simulink model "simulator"  (R2022b)
settings: Solver=FixedStepAuto  StartTime=0.0  StopTime=1800  FixedStep=1/7000  RelTol=1e-7
undefined symbols (not defined in the file): simdb
libraries: sim_lib x40, simulink_extras x15, matrix_library x9, simulink x1
(part 1 of 3)
settings Model: SimulationMode=accelerator  Creator=David  LastModifiedBy=David

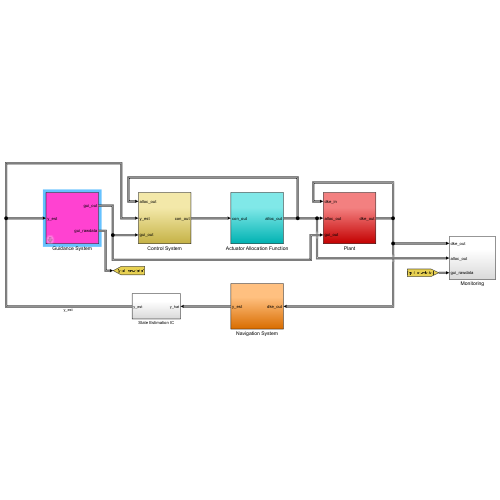
[thumbnail: Simulink's stored preview of the top-level diagram]
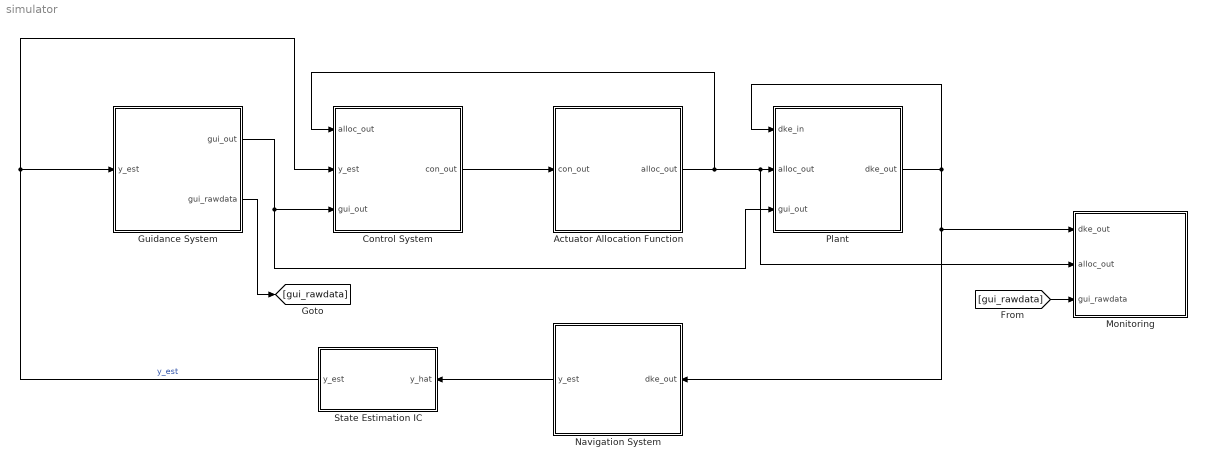
== system simulator ==
  Actuator Allocation Function : Subsystem
  Control System : Subsystem
  Guidance System : Subsystem  mask{gui=simdb.gui}
      mask prompts: gui "Guidance Parameters"
  Monitoring : Subsystem
  Navigation System : Subsystem
  Plant : Subsystem
  State Estimation IC : Subsystem
  wires:
  State Estimation IC/1(y_est) -> Control System/2(y_est), Guidance System/1(y_est)  "y_est"
  Navigation System/1(y_est) -> State Estimation IC/1(y_hat)
  Plant/1(dke_out) -> Navigation System/1(dke_out), Monitoring/1(dke_out), Plant/1(dke_in)
  Actuator Allocation Function/1(alloc_out) -> Plant/2(alloc_out), Monitoring/2(alloc_out), Control System/1(alloc_out)
  Guidance System/1(gui_out) -> Plant/3(gui_out), Control System/3(gui_out)
  Control System/1(con_out) -> Actuator Allocation Function/1(con_out)
  Guidance System/2(gui_rawdata) -> [gui_rawdata]
  [gui_rawdata] -> Monitoring/3(gui_rawdata)

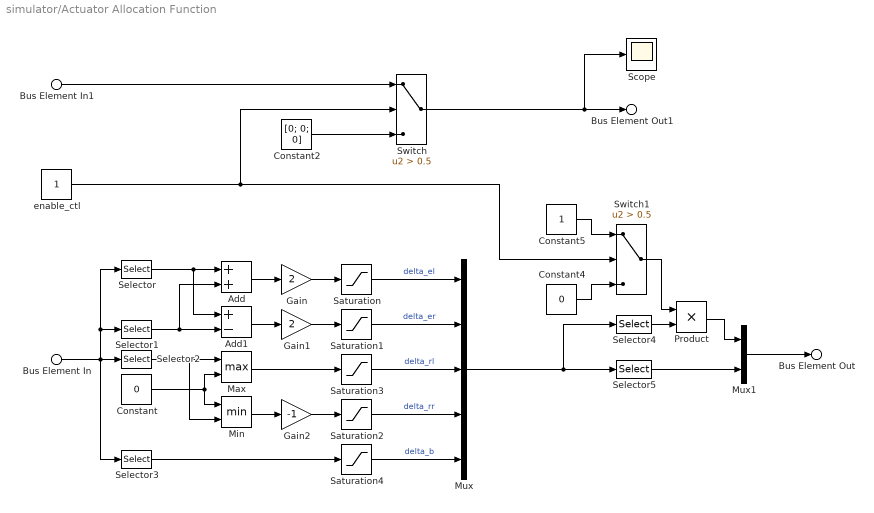
== system simulator/Actuator Allocation Function ==
  Bus Element In : Inport  PortName=con_out  Element=sc_delta_ae_cmd
  Bus Element In1 : Inport  PortName=con_out  Element=sc_rcs_tor_bod_cmd
  Add : Sum
  Add1 : Sum  Inputs=+-
  Constant : Constant  Value=0
  Constant2 : Constant  Value=[0; 0; 0]
  Constant4 : Constant  Value=0
  Constant5 : Constant
  Gain : Gain  Gain=2
  Gain1 : Gain  Gain=2
  Gain2 : Gain  Gain=-1
  Max : MinMax  Function=max  Inputs=2
  Min : MinMax  Inputs=2
  Mux : Mux  Inputs=5
  Mux1 : Mux  Inputs=2
  Product : Product
  Saturation : Saturate  UpperLimit=simdb.sc.delta_e_bounds(2)  LowerLimit=simdb.sc.delta_e_bounds(1)
  Saturation1 : Saturate  UpperLimit=simdb.sc.delta_e_bounds(2)  LowerLimit=simdb.sc.delta_e_bounds(1)
  Saturation2 : Saturate  UpperLimit=simdb.sc.delta_r_bounds(2)  LowerLimit=simdb.sc.delta_r_bounds(1)
  Saturation3 : Saturate  UpperLimit=simdb.sc.delta_r_bounds(2)  LowerLimit=simdb.sc.delta_r_bounds(1)
  Saturation4 : Saturate  UpperLimit=simdb.sc.delta_b_bounds(2)  LowerLimit=simdb.sc.delta_b_bounds(1)
  Scope : Scope
  Selector : Selector  InputPortWidth=4  IndexOptions=Index vector (dialog)  Indices=[1]  OutputSizes=1
  Selector1 : Selector  InputPortWidth=4  IndexOptions=Index vector (dialog)  Indices=[2]  OutputSizes=1
  Selector2 : Selector  InputPortWidth=4  IndexOptions=Index vector (dialog)  Indices=[3]  OutputSizes=1
  Selector3 : Selector  InputPortWidth=4  IndexOptions=Index vector (dialog)  Indices=[4]  OutputSizes=1
  Selector4 : Selector  InputPortWidth=5  IndexOptions=Index vector (dialog)  Indices=1:4  OutputSizes=1
  Selector5 : Selector  InputPortWidth=5  IndexOptions=Index vector (dialog)  Indices=[5]  OutputSizes=1
  Switch : Switch  Criteria=u2 > Threshold  Threshold=0.5  SaturateOnIntegerOverflow=off  InputSameDT=off
  Switch1 : Switch  Criteria=u2 > Threshold  Threshold=0.5  SaturateOnIntegerOverflow=off  InputSameDT=off
  enable_ctl : Constant
  Bus Element Out : Outport  PortName=alloc_out  Element=delta_ae_cmd
  Bus Element Out1 : Outport  PortName=alloc_out  Element=T_cmd
  wires:
  Bus Element In/1 -> Selector/1, Selector1/1, Selector3/1, Selector2/1
  Selector1/1 -> Add/2, Add1/2
  Selector/1 -> Add1/1, Add/1
  Add/1 -> Gain/1
  Add1/1 -> Gain1/1
  Gain/1 -> Saturation/1
  Gain1/1 -> Saturation1/1
  Selector2/1 -> Min/2, Max/1
  Constant/1 -> Max/2, Min/1
  Min/1 -> Gain2/1
  Gain2/1 -> Saturation2/1
  Max/1 -> Saturation3/1
  Selector3/1 -> Saturation4/1
  Saturation3/1 -> Mux/3  "delta_rl"
  Saturation/1 -> Mux/1  "delta_el"
  Saturation1/1 -> Mux/2  "delta_er"
  Saturation2/1 -> Mux/4  "delta_rr"
  Saturation4/1 -> Mux/5  "delta_b"
  Mux/1 -> Selector5/1, Selector4/1
  enable_ctl/1 -> Switch/2, Switch1/2
  Bus Element In1/1 -> Switch/1
  Constant2/1 -> Switch/3
  Constant4/1 -> Switch1/3
  Constant5/1 -> Switch1/1
  Selector4/1 -> Product/2
  Switch1/1 -> Product/1
  Product/1 -> Mux1/1
  Selector5/1 -> Mux1/2
  Mux1/1 -> Bus Element Out/1
  Switch/1 -> Scope/1, Bus Element Out1/1

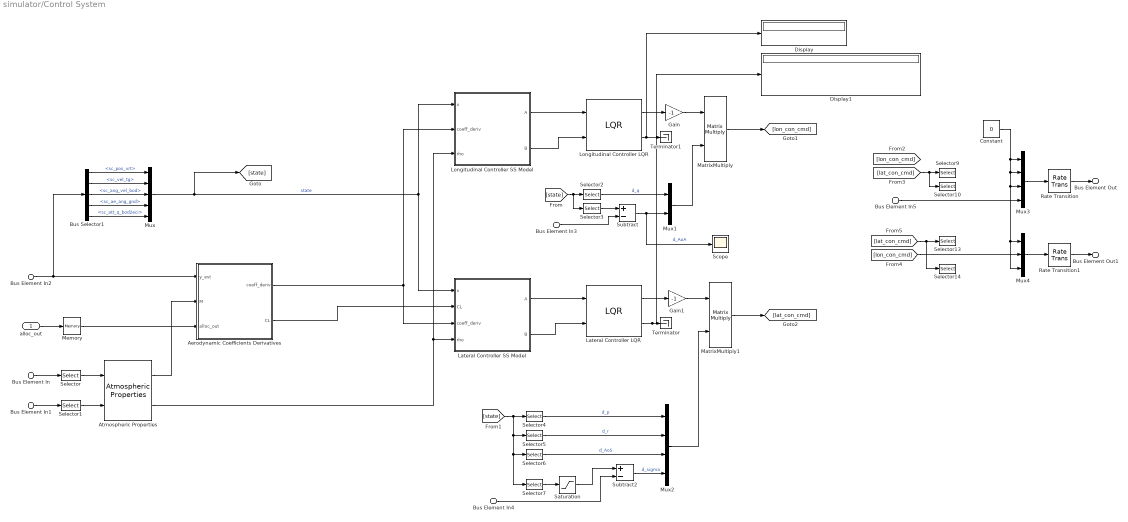
== system simulator/Control System ==
  alloc_out : Inport
  Bus Element In2 : Inport  Port=2  PortName=y_est
  Bus Element In : Inport  Port=2  PortName=y_est  Element=sc_vel_tg
  Bus Element In1 : Inport  Port=2  PortName=y_est  Element=sc_pos_vrt
  Bus Element In3 : Inport  Port=3  PortName=gui_out  Element=AoA_cmd
  Bus Element In5 : Inport  Port=3  PortName=gui_out  Element=delta_b_cmd
  Bus Element In4 : Inport  Port=3  PortName=gui_out  Element=bank_ang_cmd
  Aerodynamic Coefficients Derivatives : Subsystem
  Atmospheric Properties : sim_lib/Atmospheric Properties  Rp=simdb.env.Rp  Rg=simdb.env.Rg  gamma=simdb.env.gamma  h_base=simdb.env.h_base  T_base=simdb.env.T_base  rho_base=simdb.env.rho_base
  Bus Selector1 : BusSelector  OutputSignals=sc_pos_vrt,sc_vel_tg,sc_ang_vel_bod,sc_ae_ang_gnd,sc_att_q_bod2eci
  Constant : Constant  Value=0
  Display : Display
  Display1 : Display
  Gain : Gain  Gain=-1
  Gain1 : Gain  Gain=-1
  Lateral Controller LQR : sim_lib/LQR  Q=simdb.ctl.Q_lat  R=simdb.ctl.R_lat  X0=eye(4)
  Lateral Controller SS Model : MATLAB Function  TreatAsAtomicUnit=on  mask{S=simdb.sc.Sref, b=simdb.sc.bref, Ixx=simdb.sc.I(1,1), Izz=simdb.sc.I(3,3), m=simdb.sc.m, mu=simdb.env.mu}
      mask prompts: S "Reference area [m^2]:"; b "Lateral reference length [m]:"; Ixx "Inertia, x axis [kg*m^2]:"; Izz "Inertia, z axis [kg*m^2]:"; m "Mass [kg]:"; mu "Gravitational parameter [m^3/s^2]:"
  Longitudinal Controller LQR : sim_lib/LQR  Q=simdb.ctl.Q_lon  R=simdb.ctl.R_lon  X0=eye(2)
  Longitudinal Controller SS Model : MATLAB Function  TreatAsAtomicUnit=on  mask{S=simdb.sc.Sref, c=simdb.sc.cref, Iyy=simdb.sc.I(2,2), m=simdb.sc.m}
      mask prompts: S "Reference area [m^2]:"; c "Longitudinal reference length [m]:"; Iyy "Inertia, y axis [kg*m^2]:"; m "Mass [kg]:"
  MatrixMultiply : Product  Multiplication=Matrix(*)
  MatrixMultiply1 : Product  Multiplication=Matrix(*)
  Memory : Memory
  Mux : Mux  Inputs=5
  Mux1 : Mux  Inputs=2
  Mux2 : Mux
  Mux3 : Mux
  Mux4 : Mux  Inputs=3
  Rate Transition : RateTransition  InitialCondition=[0; 0; 0; 0]  OutPortSampleTime=simdb.ctl.tsamp
  Rate Transition1 : RateTransition  InitialCondition=[0; 0; 0]  OutPortSampleTime=simdb.ctl.tsamp
  Saturation : Saturate  UpperLimit=deg2rad(180)  LowerLimit=deg2rad(-180)
  Scope : Scope
  Selector : Selector  InputPortWidth=3  IndexOptions=Index vector (dialog)  Indices=[1]  OutputSizes=1
  Selector1 : Selector  InputPortWidth=3  IndexOptions=Index vector (dialog)  Indices=[1]  OutputSizes=1
  Selector10 : Selector  InputPortWidth=4  IndexOptions=Index vector (dialog)  Indices=[2]  OutputSizes=1
  Selector13 : Selector  InputPortWidth=4  IndexOptions=Index vector (dialog)  Indices=[3]  OutputSizes=1
  Selector14 : Selector  InputPortWidth=4  IndexOptions=Index vector (dialog)  Indices=[4]  OutputSizes=1
  Selector2 : Selector  InputPortWidth=16  IndexOptions=Index vector (dialog)  Indices=[8]  OutputSizes=1
  Selector3 : Selector  InputPortWidth=16  IndexOptions=Index vector (dialog)  Indices=[10]  OutputSizes=1
  Selector4 : Selector  InputPortWidth=16  IndexOptions=Index vector (dialog)  Indices=[7]  OutputSizes=1
  Selector5 : Selector  InputPortWidth=16  IndexOptions=Index vector (dialog)  Indices=[9]  OutputSizes=1
  Selector6 : Selector  InputPortWidth=16  IndexOptions=Index vector (dialog)  Indices=[9]  OutputSizes=1
  Selector7 : Selector  InputPortWidth=16  IndexOptions=Index vector (dialog)  Indices=[9]  OutputSizes=1
  Selector9 : Selector  InputPortWidth=4  IndexOptions=Index vector (dialog)  Indices=[1]  OutputSizes=1
  Subtract : Sum  Inputs=+-
  Subtract2 : Sum  Inputs=+-
  Terminator : Terminator
  Terminator1 : Terminator
  Bus Element Out : Outport  PortName=con_out  Element=sc_delta_ae_cmd
  Bus Element Out1 : Outport  PortName=con_out  Element=sc_rcs_tor_bod_cmd
  wires:
  Lateral Controller SS Model/1(A) -> Lateral Controller LQR/1
  Lateral Controller SS Model/2(B) -> Lateral Controller LQR/2
  Longitudinal Controller SS Model/1(A) -> Longitudinal Controller LQR/1
  Longitudinal Controller SS Model/2(B) -> Longitudinal Controller LQR/2
  alloc_out/1 -> Memory/1
  Memory/1 -> Aerodynamic Coefficients Derivatives/3(alloc_out)
  Selector/1 -> Atmospheric Properties/1
  Bus Element In/1 -> Selector/1
  Bus Element In1/1 -> Selector1/1
  Selector1/1 -> Atmospheric Properties/2
  Bus Element In2/1 -> Bus Selector1/1, Aerodynamic Coefficients Derivatives/1(y_est)
  Atmospheric Properties/1 -> Aerodynamic Coefficients Derivatives/2(M)
  Bus Selector1/3 -> Mux/3  "<sc_ang_vel_bod>"
  Bus Selector1/4 -> Mux/4  "<sc_ae_ang_gnd>"
  Bus Selector1/5 -> Mux/5  "<sc_att_q_bod2eci>"
  Bus Selector1/2 -> Mux/2  "<sc_vel_tg>"
  Bus Selector1/1 -> Mux/1  "<sc_pos_vrt>"
  Mux/1 -> [state], Longitudinal Controller SS Model/1(x), Lateral Controller SS Model/1(x)  "state"
  Aerodynamic Coefficients Derivatives/1(coeff_deriv) -> Longitudinal Controller SS Model/2(coeff_deriv), Lateral Controller SS Model/3(coeff_deriv)
  Atmospheric Properties/2 -> Lateral Controller SS Model/4(rho), Longitudinal Controller SS Model/3(rho)
  Lateral Controller LQR/2 -> Terminator/1, Display1/1
  Longitudinal Controller LQR/2 -> Terminator1/1, Display/1
  [state] -> Selector3/1, Selector2/1
  Selector3/1 -> Subtract/1
  Bus Element In3/1 -> Subtract/2
  Subtract/1 -> Scope/1, Mux1/2  "d_AoA"
  Selector2/1 -> Mux1/1  "d_q"
  Longitudinal Controller LQR/1 -> Gain/1
  Mux1/1 -> MatrixMultiply/2
  Gain/1 -> MatrixMultiply/1
  Lateral Controller LQR/1 -> Gain1/1
  Gain1/1 -> MatrixMultiply1/1
  [state] -> Selector7/1, Selector6/1, Selector5/1, Selector4/1
  Selector5/1 -> Mux2/2  "d_r"
  Selector4/1 -> Mux2/1  "d_p"
  Subtract2/1 -> Mux2/4  "d_sigma"
  Selector7/1 -> Saturation/1
  Selector6/1 -> Mux2/3  "d_AoS"
  Mux3/1 -> Rate Transition/1
  MatrixMultiply1/1 -> [lat_con_cmd]
  [lat_con_cmd] -> Selector10/1, Selector9/1
  Bus Element In5/1 -> Mux3/4
  Mux4/1 -> Rate Transition1/1
  [lat_con_cmd] -> Selector14/1, Selector13/1
  Aerodynamic Coefficients Derivatives/2(CL) -> Lateral Controller SS Model/2(CL)
  Mux2/1 -> MatrixMultiply1/2
  Rate Transition/1 -> Bus Element Out/1
  Rate Transition1/1 -> Bus Element Out1/1
  Bus Element In4/1 -> Subtract2/2
  Saturation/1 -> Subtract2/1
  Constant/1 -> Mux3/1, Mux4/3, Mux4/1, Mux3/3, Mux3/2
  MatrixMultiply/1 -> [lon_con_cmd]
  [lon_con_cmd] -> Mux4/2

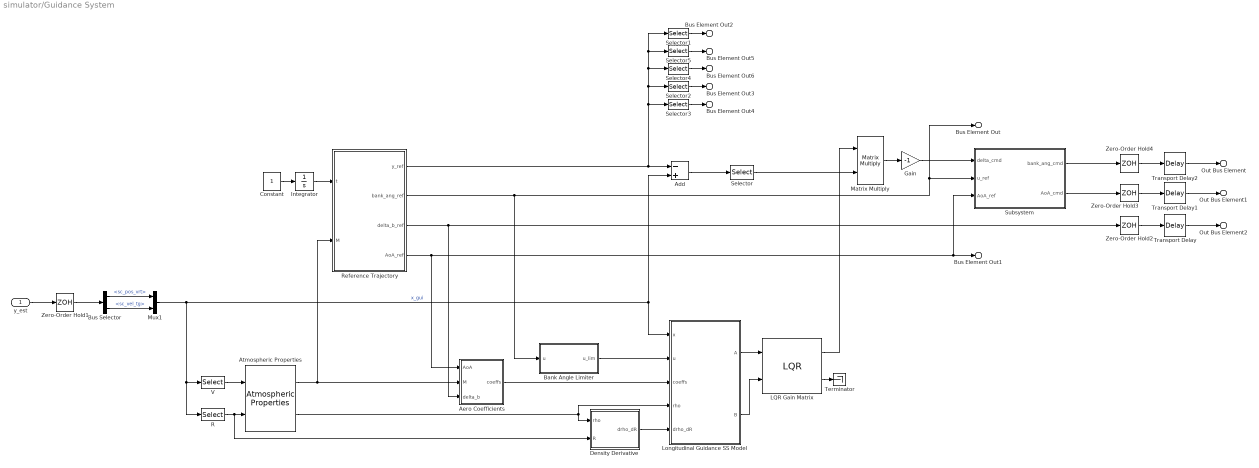
== system simulator/Guidance System ==
  y_est : Inport
  Add : Sum  Inputs=-+
  Aero Coefficients : Subsystem
  Atmospheric Properties : sim_lib/Atmospheric Properties  Rp=simdb.env.Rp  Rg=simdb.env.Rg  gamma=simdb.env.gamma  h_base=simdb.env.h_base  T_base=simdb.env.T_base  rho_base=simdb.env.rho_base
  Bank Angle Limiter : Subsystem
  Bus Selector : BusSelector  OutputSignals=sc_pos_vrt,sc_vel_tg
  Constant : Constant
  Density Derivative : Subsystem
  Gain : Gain  Gain=-1
  Integrator : Integrator  InitialCondition=1
  LQR Gain Matrix : sim_lib/LQR  Q=gui.Q  R=gui.R  X0=eye(3)
  Longitudinal Guidance SS Model : MATLAB Function  TreatAsAtomicUnit=on  mask{S=simdb.sc.Sref, m=simdb.sc.m, mu=simdb.env.mu}
      mask prompts: S "Reference area"; m "Spacecraft mass"; mu "Gravitational constant"
  Matrix Multiply : Product  Multiplication=Matrix(*)
  Mux1 : Mux  Inputs=2
  R : Selector  InputPortWidth=6  IndexOptions=Index vector (dialog)  Indices=[1]  OutputSizes=1
  Reference Trajectory : Subsystem
  Selector : Selector  InputPortWidth=6  IndexOptions=Index vector (dialog)  Indices=[1 4 5]  OutputSizes=1
  Selector1 : Selector  InputPortWidth=6  IndexOptions=Index vector (dialog)  Indices=1  OutputSizes=1
  Selector2 : Selector  InputPortWidth=6  IndexOptions=Index vector (dialog)  Indices=4  OutputSizes=1
  Selector3 : Selector  InputPortWidth=6  IndexOptions=Index vector (dialog)  Indices=5  OutputSizes=1
  Selector4 : Selector  InputPortWidth=6  IndexOptions=Index vector (dialog)  Indices=3  OutputSizes=1
  Selector5 : Selector  InputPortWidth=6  IndexOptions=Index vector (dialog)  Indices=2  OutputSizes=1
  Subsystem : Subsystem
  Terminator : Terminator
  Transport Delay : TransportDelay  DelayTime=gui.delay  BufferSize=4096
  Transport Delay1 : TransportDelay  DelayTime=gui.delay  InitialOutput=deg2rad(-40)  BufferSize=4096
  Transport Delay2 : TransportDelay  DelayTime=gui.delay  InitialOutput=deg2rad(-165)  BufferSize=4096
  V : Selector  InputPortWidth=6  IndexOptions=Index vector (dialog)  Indices=[4]  OutputSizes=1
  Zero-Order Hold{1..4} (4 alike) : ZeroOrderHold  SampleTime=gui.tsample
  Out Bus Element : Outport  PortName=gui_out  Element=bank_ang_cmd
  Out Bus Element2 : Outport  PortName=gui_out  Element=delta_b_cmd
  Out Bus Element1 : Outport  PortName=gui_out  Element=AoA_cmd
  Bus Element Out : Outport  Port=2  PortName=gui_rawdata  Element=bank_ang_ref
  Bus Element Out1 : Outport  Port=2  PortName=gui_rawdata  Element=AoA_ref
  Bus Element Out2 : Outport  Port=2  PortName=gui_rawdata  Element=R_ref
  Bus Element Out3 : Outport  Port=2  PortName=gui_rawdata  Element=V_ref
  Bus Element Out4 : Outport  Port=2  PortName=gui_rawdata  Element=gamma_ref
  Bus Element Out5 : Outport  Port=2  PortName=gui_rawdata  Element=tau_ref
  Bus Element Out6 : Outport  Port=2  PortName=gui_rawdata  Element=delta_ref
  wires:
  y_est/1 -> Zero-Order Hold1/1
  Mux1/1 -> V/1, R/1, Longitudinal Guidance SS Model/1(x), Add/2  "x_gui"
  Zero-Order Hold2/1 -> Transport Delay/1
  Constant/1 -> Integrator/1
  Longitudinal Guidance SS Model/1(A) -> LQR Gain Matrix/1
  Matrix Multiply/1 -> Gain/1
  Reference Trajectory/3(delta_b_ref) -> Aero Coefficients/3(delta_b), Zero-Order Hold2/1
  Reference Trajectory/2(bank_ang_ref) -> Bank Angle Limiter/1(u), Bus Element Out/1, Subsystem/2(u_ref)
  Reference Trajectory/4(AoA_ref) -> Aero Coefficients/1(AoA), Subsystem/3(AoA_ref), Bus Element Out1/1
  Integrator/1 -> Reference Trajectory/1(t)
  Selector/1 -> Matrix Multiply/2
  Add/1 -> Selector/1
  Atmospheric Properties/2 -> Density Derivative/1(rho), Longitudinal Guidance SS Model/4(rho)
  Atmospheric Properties/1 -> Aero Coefficients/2(M), Reference Trajectory/2(M)
  V/1 -> Atmospheric Properties/1
  R/1 -> Density Derivative/2(R), Atmospheric Properties/2
  Density Derivative/1(drho_dR) -> Longitudinal Guidance SS Model/5(drho_dR)
  Longitudinal Guidance SS Model/2(B) -> LQR Gain Matrix/2
  LQR Gain Matrix/1 -> Matrix Multiply/1
  LQR Gain Matrix/2 -> Terminator/1
  Zero-Order Hold1/1 -> Bus Selector/1
  Bus Selector/1 -> Mux1/1  "<sc_pos_vrt>"
  Bus Selector/2 -> Mux1/2  "<sc_vel_tg>"
  Transport Delay/1 -> Out Bus Element2/1
  Zero-Order Hold4/1 -> Transport Delay2/1
  Transport Delay2/1 -> Out Bus Element/1
  Aero Coefficients/1(coeffs) -> Longitudinal Guidance SS Model/3(coeffs)
  Gain/1 -> Subsystem/1(delta_cmd)
  Subsystem/1(bank_ang_cmd) -> Zero-Order Hold4/1
  Transport Delay1/1 -> Out Bus Element1/1
  Zero-Order Hold3/1 -> Transport Delay1/1
  Subsystem/2(AoA_cmd) -> Zero-Order Hold3/1
  Bank Angle Limiter/1(u_lim) -> Longitudinal Guidance SS Model/2(u)
  Selector1/1 -> Bus Element Out2/1
  Selector2/1 -> Bus Element Out3/1
  Selector3/1 -> Bus Element Out4/1
  Selector4/1 -> Bus Element Out6/1
  Reference Trajectory/1(y_ref) -> Selector4/1, Selector5/1, Selector1/1, Selector2/1, Selector3/1, Add/1
  Selector5/1 -> Bus Element Out5/1

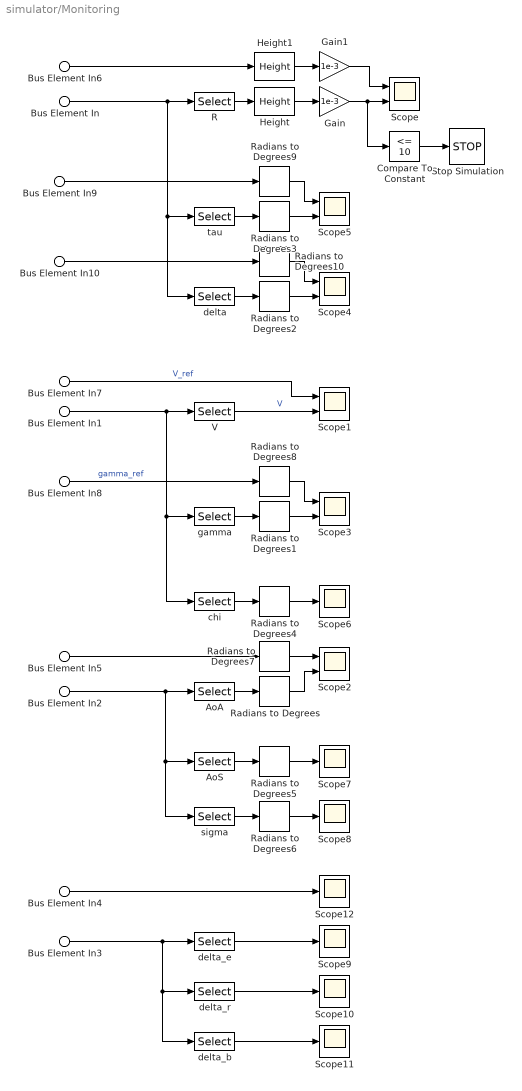
== system simulator/Monitoring ==
  Bus Element In : Inport  PortName=dke_out  Element=sc_pos_vrt
  Bus Element In1 : Inport  PortName=dke_out  Element=sc_vel_tg
  Bus Element In2 : Inport  PortName=dke_out  Element=sc_ae_ang_gnd
  Bus Element In4 : Inport  PortName=dke_out  Element=sc_att_q_bod2eci
  Bus Element In3 : Inport  Port=2  PortName=alloc_out  Element=delta_ae_cmd
  Bus Element In5 : Inport  Port=3  PortName=gui_rawdata  Element=AoA_ref
  Bus Element In6 : Inport  Port=3  PortName=gui_rawdata  Element=R_ref
  Bus Element In7 : Inport  Port=3  PortName=gui_rawdata  Element=V_ref
  Bus Element In8 : Inport  Port=3  PortName=gui_rawdata  Element=gamma_ref
  Bus Element In10 : Inport  Port=3  PortName=gui_rawdata  Element=delta_ref
  Bus Element In9 : Inport  Port=3  PortName=gui_rawdata  Element=tau_ref
  AoA : Selector  InputPortWidth=3  IndexOptions=Index vector (dialog)  Indices=[1]  OutputSizes=1
  AoS : Selector  InputPortWidth=3  IndexOptions=Index vector (dialog)  Indices=[2]  OutputSizes=1
  Compare To Constant : simulink/Logic and Bit Operations/Compare To Constant  relop=<=  const=10  OutDataTypeStr=boolean
  Gain : Gain  Gain=1e-3
  Gain1 : Gain  Gain=1e-3
  Height : sim_lib/Height  Rp=simdb.env.Rp
  Height1 : sim_lib/Height  Rp=simdb.env.Rp
  R : Selector  InputPortWidth=3  IndexOptions=Index vector (dialog)  Indices=[1]  OutputSizes=1
  Radians to Degrees{,1..10} (11 alike) : simulink_extras/Transformations/Radians to Degrees
  Scope{,1..5} (6 alike) : Scope  NumInputPorts=2
  Scope{6..12} (7 alike) : Scope
  Stop Simulation : Stop
  V : Selector  InputPortWidth=3  IndexOptions=Index vector (dialog)  Indices=[1]  OutputSizes=1
  chi : Selector  InputPortWidth=3  IndexOptions=Index vector (dialog)  Indices=[3]  OutputSizes=1
  delta : Selector  InputPortWidth=3  IndexOptions=Index vector (dialog)  Indices=[3]  OutputSizes=1
  delta_b : Selector  InputPortWidth=5  IndexOptions=Index vector (dialog)  Indices=[5]  OutputSizes=1
  delta_e : Selector  InputPortWidth=5  IndexOptions=Index vector (dialog)  Indices=[1 2]  OutputSizes=1
  delta_r : Selector  InputPortWidth=5  IndexOptions=Index vector (dialog)  Indices=[3 4]  OutputSizes=1
  gamma : Selector  InputPortWidth=3  IndexOptions=Index vector (dialog)  Indices=[2]  OutputSizes=1
  sigma : Selector  InputPortWidth=3  IndexOptions=Index vector (dialog)  Indices=[3]  OutputSizes=1
  tau : Selector  InputPortWidth=3  IndexOptions=Index vector (dialog)  Indices=[2]  OutputSizes=1
  wires:
  R/1 -> Height/1
  AoA/1 -> Radians to Degrees/1
  gamma/1 -> Radians to Degrees1/1
  Height/1 -> Gain/1
  Gain/1 -> Scope/2, Compare To Constant/1
  Compare To Constant/1 -> Stop Simulation/1
  chi/1 -> Radians to Degrees4/1
  Radians to Degrees4/1 -> Scope6/1
  tau/1 -> Radians to Degrees3/1
  delta/1 -> Radians to Degrees2/1
  Bus Element In/1 -> delta/1, tau/1, R/1
  Bus Element In1/1 -> chi/1, gamma/1, V/1
  Bus Element In2/1 -> sigma/1, AoS/1, AoA/1
  Radians to Degrees5/1 -> Scope7/1
  AoS/1 -> Radians to Degrees5/1
  Radians to Degrees6/1 -> Scope8/1
  sigma/1 -> Radians to Degrees6/1
  Bus Element In3/1 -> delta_b/1, delta_r/1, delta_e/1
  delta_e/1 -> Scope9/1
  delta_r/1 -> Scope10/1
  delta_b/1 -> Scope11/1
  Bus Element In4/1 -> Scope12/1
  Bus Element In5/1 -> Radians to Degrees7/1
  Radians to Degrees7/1 -> Scope2/1
  Radians to Degrees/1 -> Scope2/2
  Height1/1 -> Gain1/1
  Bus Element In6/1 -> Height1/1
  Gain1/1 -> Scope/1
  V/1 -> Scope1/2  "V"
  Bus Element In7/1 -> Scope1/1  "V_ref"
  Bus Element In8/1 -> Radians to Degrees8/1  "gamma_ref"
  Radians to Degrees8/1 -> Scope3/1
  Radians to Degrees1/1 -> Scope3/2
  Radians to Degrees3/1 -> Scope5/2
  Bus Element In9/1 -> Radians to Degrees9/1
  Radians to Degrees2/1 -> Scope4/2
  Bus Element In10/1 -> Radians to Degrees10/1
  Radians to Degrees9/1 -> Scope5/1
  Radians to Degrees10/1 -> Scope4/1

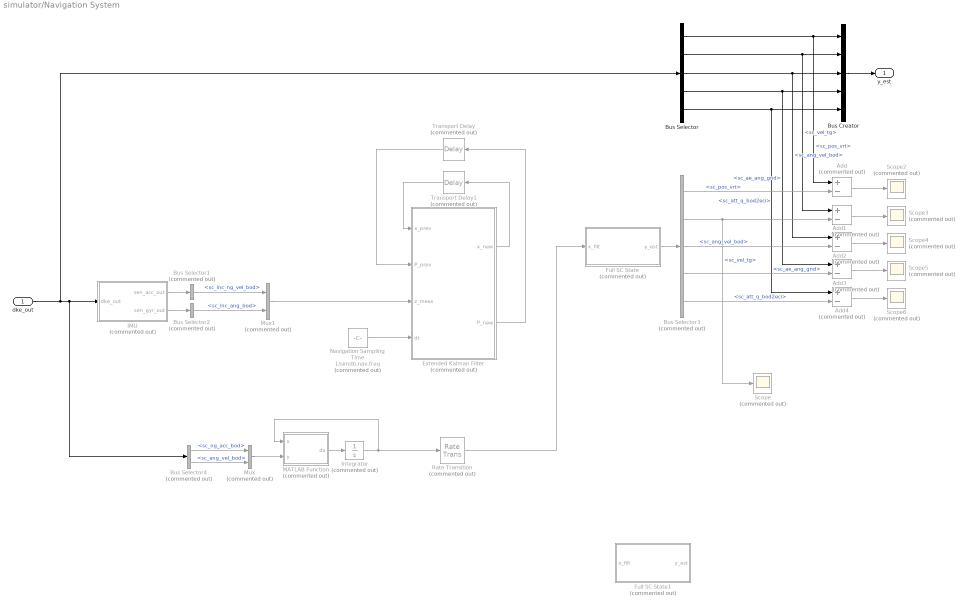
== system simulator/Navigation System ==
  dke_out : Inport
  Add{,1..4} (5 alike) : Sum  Commented=on  Inputs=+-
  Bus Creator : BusCreator  Inputs=5
  Bus Selector : BusSelector  OutputSignals=sc_pos_vrt,sc_vel_tg,sc_ang_vel_bod,sc_ae_ang_gnd,sc_att_q_bod2eci
  Bus Selector1 : BusSelector  Commented=on  OutputSignals=sc_inc_ng_vel_bod
  Bus Selector2 : BusSelector  Commented=on  OutputSignals=sc_inc_ang_bod
  Bus Selector3 : BusSelector  Commented=on  OutputSignals=sc_pos_vrt,sc_vel_tg,sc_ang_vel_bod,sc_ae_ang_gnd,sc_att_q_bod2eci
  Bus Selector4 : BusSelector  Commented=on  OutputSignals=sc_ng_acc_bod,sc_ang_vel_bod
  Extended Kalman Filter : Subsystem  Commented=on
  Full SC State : Subsystem  Commented=on
  Full SC State1 : Subsystem  Commented=on
  IMU : Subsystem  Commented=on  mask{gyr=simdb.gyr, acc=simdb.acc}
      mask prompts: gyr "GYR Parameters"; acc "ACC Parameters"
  Integrator : Integrator  Commented=on  InitialCondition=simdb.nav.x0
  MATLAB Function : MATLAB Function  Commented=on  TreatAsAtomicUnit=on  mask{mu=simdb.env.mu, K=simdb.nav.dq_K}
  Mux : Mux  Commented=on  Inputs=2
  Mux1 : Mux  Commented=on  Inputs=2
  Navigation Sampling Time : Constant  Commented=on  Value=1/simdb.nav.freq
  Rate Transition : RateTransition  Commented=on  InitialCondition=simdb.nav.x0  OutPortSampleTime=simdb.nav.tsamp
  Scope{,2..6} (6 alike) : Scope  Commented=on
  Transport Delay : TransportDelay  Commented=on  DelayTime=simdb.nav.tsamp  InitialOutput=simdb.nav.P0
  Transport Delay1 : TransportDelay  Commented=on  DelayTime=simdb.nav.tsamp  InitialOutput=simdb.nav.x0
  y_est : Outport
  wires:
  IMU/1(sen_acc_out) -> Bus Selector1/1
  IMU/2(sen_gyr_out) -> Bus Selector2/1
  Bus Selector1/1 -> Mux1/1  "<sc_inc_ng_vel_bod>"
  Bus Selector2/1 -> Mux1/2  "<sc_inc_ang_bod>"
  dke_out/1 -> Bus Selector/1, Bus Selector4/1, IMU/1(dke_out)
  Transport Delay/1 -> Extended Kalman Filter/2(P_prev)
  Extended Kalman Filter/2(P_new) -> Transport Delay/1
  Transport Delay1/1 -> Extended Kalman Filter/1(x_prev)
  Navigation Sampling Time/1 -> Extended Kalman Filter/4(dt)
  Mux1/1 -> Extended Kalman Filter/3(z_meas)
  Extended Kalman Filter/1(x_new) -> Transport Delay1/1
  Bus Selector/5 -> Add4/1, Bus Creator/5  "<sc_att_q_bod2eci>"
  Bus Selector/4 -> Add3/1, Bus Creator/4  "<sc_ae_ang_gnd>"
  Bus Selector/3 -> Add2/1, Bus Creator/3  "<sc_ang_vel_bod>"
  Bus Selector/2 -> Add1/1, Bus Creator/2  "<sc_vel_tg>"
  Bus Selector/1 -> Add/1, Bus Creator/1  "<sc_pos_vrt>"
  Bus Creator/1 -> y_est/1
  Full SC State/1(y_est) -> Bus Selector3/1
  Bus Selector3/1 -> Add/2  "<sc_pos_vrt>"
  Bus Selector3/2 -> Scope/1, Add1/2  "<sc_vel_tg>"
  Bus Selector3/5 -> Add4/2  "<sc_att_q_bod2eci>"
  Bus Selector3/4 -> Add3/2  "<sc_ae_ang_gnd>"
  Bus Selector3/3 -> Add2/2  "<sc_ang_vel_bod>"
  Add/1 -> Scope2/1
  Add1/1 -> Scope3/1
  Add2/1 -> Scope4/1
  Add3/1 -> Scope5/1
  Add4/1 -> Scope6/1
  MATLAB Function/1(dx) -> Integrator/1
  Integrator/1 -> Rate Transition/1, MATLAB Function/1(x)
  Bus Selector4/1 -> Mux/1  "<sc_ng_acc_bod>"
  Bus Selector4/2 -> Mux/2  "<sc_ang_vel_bod>"
  Mux/1 -> MATLAB Function/2(y)
  Rate Transition/1 -> Full SC State/1(x_filt)

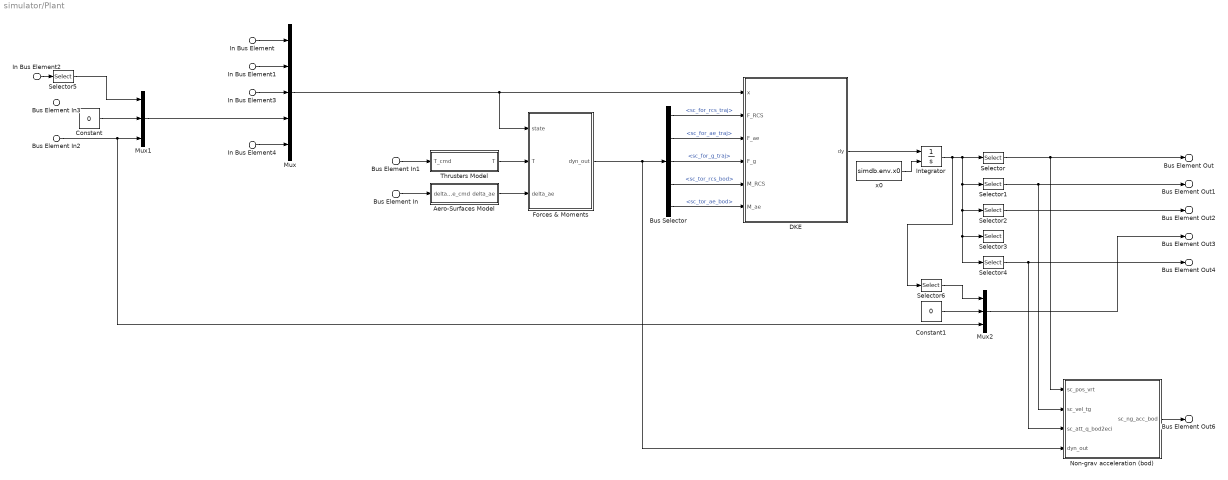
== system simulator/Plant ==
  In Bus Element : Inport  PortName=dke_in  Element=sc_pos_vrt
  In Bus Element1 : Inport  PortName=dke_in  Element=sc_vel_tg
  In Bus Element3 : Inport  PortName=dke_in  Element=sc_ang_vel_bod
  In Bus Element4 : Inport  PortName=dke_in  Element=sc_att_q_bod2eci
  In Bus Element2 : Inport  PortName=dke_in  Element=sc_ae_ang_gnd
  Bus Element In : Inport  Port=2  PortName=alloc_out  Element=delta_ae_cmd
  Bus Element In1 : Inport  Port=2  PortName=alloc_out  Element=T_cmd
  Bus Element In2 : Inport  Port=3  PortName=gui_out  Element=bank_ang_cmd
  Bus Element In3 : Inport  Port=3  PortName=gui_out  Element=AoA_cmd
  Aero-Surfaces Model : Subsystem
  Bus Selector : BusSelector  OutputSignals=sc_for_rcs_traj,sc_for_ae_traj,sc_for_g_traj,sc_tor_rcs_bod,sc_tor_ae_bod
  Constant : Constant  Value=0
  Constant1 : Constant  Value=0
  DKE : MATLAB Function  TreatAsAtomicUnit=on  mask{m=simdb.sc.m, omega_cb=simdb.env.omega_cb, I=simdb.sc.I}
  Forces & Moments : Subsystem
  Integrator : Integrator  InitialConditionSource=external
  Mux : Mux  Inputs=5
  Mux1 : Mux  Inputs=3
  Mux2 : Mux  Inputs=3
  Non-grav acceleration (bod) : Subsystem
  Selector : Selector  InputPortWidth=16  IndexOptions=Index vector (dialog)  Indices=[1 2 3]  OutputSizes=1
  Selector1 : Selector  InputPortWidth=16  IndexOptions=Index vector (dialog)  Indices=[4 5 6]  OutputSizes=1
  Selector2 : Selector  InputPortWidth=16  IndexOptions=Index vector (dialog)  Indices=[7 8 9]  OutputSizes=1
  Selector3 : Selector  InputPortWidth=16  IndexOptions=Index vector (dialog)  Indices=[10 11 12]  OutputSizes=1
  Selector4 : Selector  InputPortWidth=16  IndexOptions=Index vector (dialog)  Indices=[13 14 15 16]  OutputSizes=1
  Selector5 : Selector  InputPortWidth=3  IndexOptions=Index vector (dialog)  Indices=1  OutputSizes=1
  Selector6 : Selector  InputPortWidth=16  IndexOptions=Index vector (dialog)  Indices=10  OutputSizes=1
  Thrusters Model : Subsystem
  x0 : Constant  Value=simdb.env.x0
  Bus Element Out : Outport  PortName=dke_out  Element=sc_pos_vrt
  Bus Element Out1 : Outport  PortName=dke_out  Element=sc_vel_tg
  Bus Element Out2 : Outport  PortName=dke_out  Element=sc_ang_vel_bod
  Bus Element Out3 : Outport  PortName=dke_out  Element=sc_ae_ang_gnd
  Bus Element Out4 : Outport  PortName=dke_out  Element=sc_att_q_bod2eci
  Bus Element Out6 : Outport  PortName=dke_out  Element=sc_ng_acc_bod
  wires:
  Thrusters Model/1(T) -> Forces & Moments/2(T)
  Aero-Surfaces Model/1(delta_ae) -> Forces & Moments/3(delta_ae)
  Mux/1 -> Forces & Moments/1(state), DKE/1(x)
  DKE/1(dy) -> Integrator/1
  x0/1 -> Integrator/2
  Selector/1 -> Bus Element Out/1, Non-grav acceleration (bod)/1(sc_pos_vrt)
  Selector1/1 -> Bus Element Out1/1, Non-grav acceleration (bod)/2(sc_vel_tg)
  Selector2/1 -> Bus Element Out2/1
  Selector4/1 -> Bus Element Out4/1, Non-grav acceleration (bod)/3(sc_att_q_bod2eci)
  Integrator/1 -> Selector6/1, Selector4/1, Selector3/1, Selector2/1, Selector1/1, Selector/1
  Forces & Moments/1(dyn_out) -> Non-grav acceleration (bod)/4(dyn_out), Bus Selector/1
  Bus Selector/1 -> DKE/2(F_RCS)  "<sc_for_rcs_traj>"
  Bus Selector/2 -> DKE/3(F_ae)  "<sc_for_ae_traj>"
  Bus Selector/3 -> DKE/4(F_g)  "<sc_for_g_traj>"
  Bus Selector/4 -> DKE/5(M_RCS)  "<sc_tor_rcs_bod>"
  Bus Selector/5 -> DKE/6(M_ae)  "<sc_tor_ae_bod>"
  Non-grav acceleration (bod)/1(sc_ng_acc_bod) -> Bus Element Out6/1
  In Bus Element/1 -> Mux/1
  In Bus Element1/1 -> Mux/2
  In Bus Element4/1 -> Mux/5
  Bus Element In1/1 -> Thrusters Model/1(T_cmd)
  In Bus Element2/1 -> Selector5/1
  Constant/1 -> Mux1/2
  Bus Element In2/1 -> Mux2/3, Mux1/3
  Bus Element In/1 -> Aero-Surfaces Model/1(delta_ae_cmd)
  Constant1/1 -> Mux2/2
  Mux2/1 -> Bus Element Out3/1
  Mux1/1 -> Mux/4
  In Bus Element3/1 -> Mux/3
  Selector6/1 -> Mux2/1
  Selector5/1 -> Mux1/1

== system simulator/State Estimation IC ==
  y_hat : Inport
  Bus Creator : BusCreator  Inputs=5
  Bus Selector : BusSelector  OutputSignals=sc_pos_vrt,sc_vel_tg,sc_ang_vel_bod,sc_ae_ang_gnd,sc_att_q_bod2eci
  IC : InitialCondition  Value=simdb.nav.sc_pos_vrt_init
  IC1 : InitialCondition  Value=simdb.nav.sc_vel_tg_init
  IC2 : InitialCondition  Value=simdb.nav.sc_ang_vel_bod_init
  IC3 : InitialCondition  Value=simdb.nav.sc_ae_ang_gnd_init
  IC4 : InitialCondition  Value=simdb.nav.sc_att_q_bod2eci_init
  y_est : Outport
  wires:
  Bus Selector/3 -> IC2/1  "<sc_ang_vel_bod>"
  Bus Selector/1 -> IC/1  "<sc_pos_vrt>"
  IC4/1 -> Bus Creator/5  "sc_att_q_bod2eci"
  Bus Selector/2 -> IC1/1  "<sc_vel_tg>"
  Bus Selector/4 -> IC3/1  "<sc_ae_ang_gnd>"
  Bus Selector/5 -> IC4/1  "<sc_att_q_bod2eci>"
  Bus Creator/1 -> y_est/1
  IC/1 -> Bus Creator/1  "sc_pos_vrt"
  IC3/1 -> Bus Creator/4  "sc_ae_ang_gnd"
  IC1/1 -> Bus Creator/2  "sc_vel_tg"
  IC2/1 -> Bus Creator/3  "sc_ang_vel_bod"
  y_hat/1 -> Bus Selector/1

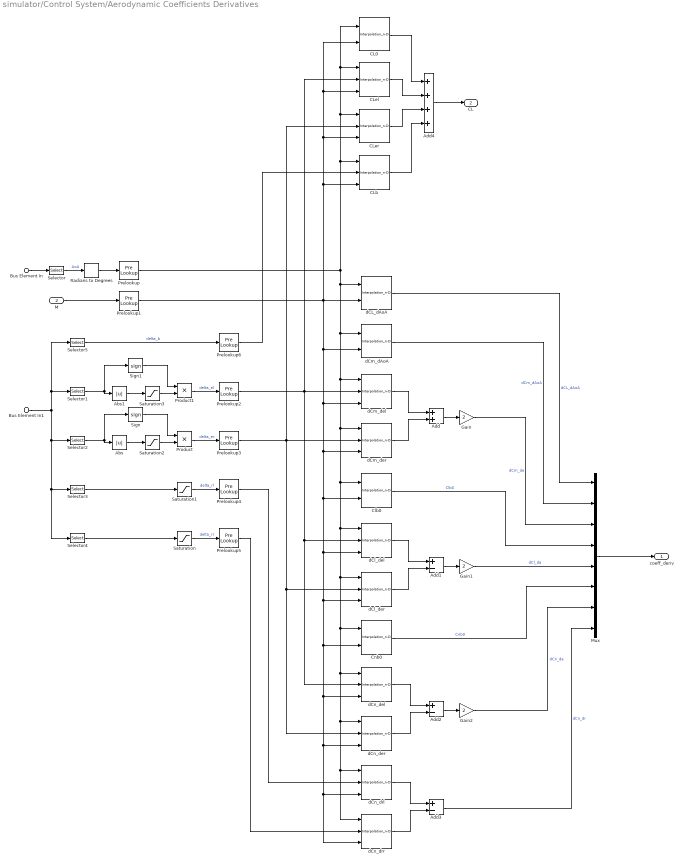
== system simulator/Control System/Aerodynamic Coefficients Derivatives ==
  Bus Element In : Inport  PortName=y_est  Element=sc_ae_ang_gnd
  M : Inport  Port=2
  Bus Element In1 : Inport  Port=3  PortName=alloc_out  Element=delta_ae_cmd
  Abs : Abs  SaturateOnIntegerOverflow=off
  Abs1 : Abs  SaturateOnIntegerOverflow=off
  Add : Sum
  Add1 : Sum  Inputs=+-
  Add2 : Sum  Inputs=+-
  Add3 : Sum  Inputs=+-
  Add4 : Sum  Inputs=++++
  CL0 : Interpolation_n-D  Table=simdb.aero.CL0  RequireIndexFractionAsBus=on  RemoveProtectionIndex=on  InternalRulePriority=Speed
      settings: InputPortMap=u0,u1
  CLb : Interpolation_n-D  NumberOfTableDimensions=3  Table=simdb.aero.CLb  RequireIndexFractionAsBus=on  RemoveProtectionIndex=on  InternalRulePriority=Speed
      settings: InputPortMap=u0,u1,u2
  CLel : Interpolation_n-D  NumberOfTableDimensions=3  Table=simdb.aero.CLel  RequireIndexFractionAsBus=on  RemoveProtectionIndex=on  InternalRulePriority=Speed
      settings: InputPortMap=u0,u1,u2
  CLer : Interpolation_n-D  NumberOfTableDimensions=3  Table=simdb.aero.CLel  RequireIndexFractionAsBus=on  RemoveProtectionIndex=on  InternalRulePriority=Speed
      settings: InputPortMap=u0,u1,u2
  Clb0 : Interpolation_n-D  Table=simdb.aero.Clb0  RequireIndexFractionAsBus=on  RemoveProtectionIndex=on  InternalRulePriority=Speed
      settings: InputPortMap=u0,u1
  Cnb0 : Interpolation_n-D  Table=simdb.aero.Cnb0  RequireIndexFractionAsBus=on  RemoveProtectionIndex=on  InternalRulePriority=Speed
      settings: InputPortMap=u0,u1
  Gain : Gain  Gain=2
  Gain1 : Gain  Gain=2
  Gain2 : Gain  Gain=2
  Mux : Mux  Inputs=8
  Prelookup : PreLookup  BreakpointsData=simdb.aero.AoA_table  OutputSelection=Index and fraction as bus  BeginIndexSearchUsingPreviousIndexResult=on  ExtrapMethod=Linear  RemoveProtectionInput=on
  Prelookup1 : PreLookup  BreakpointsData=simdb.aero.M_table  OutputSelection=Index and fraction as bus  BeginIndexSearchUsingPreviousIndexResult=on  ExtrapMethod=Linear  RemoveProtectionInput=on
  Prelookup2 : PreLookup  BreakpointsData=simdb.aero.delta_el_table  OutputSelection=Index and fraction as bus  BeginIndexSearchUsingPreviousIndexResult=on  ExtrapMethod=Linear  RemoveProtectionInput=on
  Prelookup3 : PreLookup  BreakpointsData=simdb.aero.delta_el_table  OutputSelection=Index and fraction as bus  BeginIndexSearchUsingPreviousIndexResult=on  ExtrapMethod=Linear  RemoveProtectionInput=on
  Prelookup4 : PreLookup  BreakpointsData=simdb.aero.delta_rl_table  OutputSelection=Index and fraction as bus  BeginIndexSearchUsingPreviousIndexResult=on  ExtrapMethod=Linear  RemoveProtectionInput=on
  Prelookup5 : PreLookup  BreakpointsData=simdb.aero.delta_rl_table  OutputSelection=Index and fraction as bus  BeginIndexSearchUsingPreviousIndexResult=on  ExtrapMethod=Linear  RemoveProtectionInput=on
  Prelookup6 : PreLookup  BreakpointsData=simdb.aero.delta_b_table  OutputSelection=Index and fraction as bus  BeginIndexSearchUsingPreviousIndexResult=on  ExtrapMethod=Linear  RemoveProtectionInput=on
  Product : Product
  Product1 : Product
  Radians to Degrees : simulink_extras/Transformations/Radians to Degrees
  Saturation : Saturate  UpperLimit=simdb.sc.delta_r_bounds(2)  LowerLimit=simdb.sc.delta_r_bounds(1)+1
  Saturation1 : Saturate  UpperLimit=simdb.sc.delta_r_bounds(2)  LowerLimit=simdb.sc.delta_r_bounds(1)+1
  Saturation2 : Saturate  UpperLimit=simdb.sc.delta_e_bounds(2)  LowerLimit=1
  Saturation3 : Saturate  UpperLimit=simdb.sc.delta_e_bounds(2)  LowerLimit=1
  Selector : Selector  InputPortWidth=3  IndexOptions=Index vector (dialog)  Indices=[1]  OutputSizes=1
  Selector1 : Selector  InputPortWidth=5  IndexOptions=Index vector (dialog)  Indices=[1]  OutputSizes=1
  Selector2 : Selector  InputPortWidth=5  IndexOptions=Index vector (dialog)  Indices=[2]  OutputSizes=1
  Selector3 : Selector  InputPortWidth=5  IndexOptions=Index vector (dialog)  Indices=[3]  OutputSizes=1
  Selector4 : Selector  InputPortWidth=5  IndexOptions=Index vector (dialog)  Indices=[4]  OutputSizes=1
  Selector5 : Selector  InputPortWidth=5  IndexOptions=Index vector (dialog)  Indices=[5]  OutputSizes=1
  Sign : Signum
  Sign1 : Signum
  dCL_dAoA : Interpolation_n-D  Table=simdb.aero.dCL_dAoA  RequireIndexFractionAsBus=on  RemoveProtectionIndex=on  InternalRulePriority=Speed
      settings: InputPortMap=u0,u1
  dCl_del : Interpolation_n-D  NumberOfTableDimensions=3  Table=simdb.aero.dCl_del  RequireIndexFractionAsBus=on  RemoveProtectionIndex=on  InternalRulePriority=Speed
      settings: InputPortMap=u0,u1,u2
  dCl_der : Interpolation_n-D  NumberOfTableDimensions=3  Table=simdb.aero.dCl_del  RequireIndexFractionAsBus=on  RemoveProtectionIndex=on  InternalRulePriority=Speed
      settings: InputPortMap=u0,u1,u2
  dCm_dAoA : Interpolation_n-D  Table=simdb.aero.dCm_dAoA  RequireIndexFractionAsBus=on  RemoveProtectionIndex=on  InternalRulePriority=Speed
      settings: InputPortMap=u0,u1
  dCm_del : Interpolation_n-D  NumberOfTableDimensions=3  Table=simdb.aero.dCm_del  RequireIndexFractionAsBus=on  RemoveProtectionIndex=on  InternalRulePriority=Speed
      settings: InputPortMap=u0,u1,u2
  dCm_der : Interpolation_n-D  NumberOfTableDimensions=3  Table=simdb.aero.dCm_del  RequireIndexFractionAsBus=on  RemoveProtectionIndex=on  InternalRulePriority=Speed
      settings: InputPortMap=u0,u1,u2
  dCn_del : Interpolation_n-D  NumberOfTableDimensions=3  Table=simdb.aero.dCn_del  RequireIndexFractionAsBus=on  RemoveProtectionIndex=on  InternalRulePriority=Speed
      settings: InputPortMap=u0,u1,u2
  dCn_der : Interpolation_n-D  NumberOfTableDimensions=3  Table=simdb.aero.dCn_del  RequireIndexFractionAsBus=on  RemoveProtectionIndex=on  InternalRulePriority=Speed
      settings: InputPortMap=u0,u1,u2
  dCn_drl : Interpolation_n-D  NumberOfTableDimensions=3  Table=simdb.aero.dCn_drl  RequireIndexFractionAsBus=on  RemoveProtectionIndex=on  InternalRulePriority=Speed
      settings: InputPortMap=u0,u1,u2
  dCn_drr : Interpolation_n-D  NumberOfTableDimensions=3  Table=simdb.aero.dCn_drl  RequireIndexFractionAsBus=on  RemoveProtectionIndex=on  InternalRulePriority=Speed
      settings: InputPortMap=u0,u1,u2
  coeff_deriv : Outport
  CL : Outport  Port=2
  wires:
  Bus Element In/1 -> Selector/1
  Selector/1 -> Radians to Degrees/1  "AoA"
  M/1 -> Prelookup1/1
  Prelookup/1 -> dCm_der/1, Clb0/1, dCl_der/1, Cnb0/1, dCn_der/1, dCn_drr/1, dCn_drl/1, dCn_del/1, dCl_del/1, dCm_del/1, dCm_dAoA/1, dCL_dAoA/1, CL0/1, CLel/1, CLer/1, CLb/1
  Prelookup1/1 -> dCm_der/3, Clb0/2, dCl_der/3, Cnb0/2, dCn_der/3, dCn_drr/3, dCn_drl/3, dCn_del/3, dCl_del/3, dCm_del/3, dCm_dAoA/2, CLer/3, CLel/3, CL0/2, CLb/3, dCL_dAoA/2
  Radians to Degrees/1 -> Prelookup/1
  Bus Element In1/1 -> Selector5/1, Selector1/1, Selector4/1, Selector3/1, Selector2/1
  Selector3/1 -> Saturation1/1
  Selector4/1 -> Saturation/1
  dCm_del/1 -> Add/1
  dCm_der/1 -> Add/2
  Add/1 -> Gain/1
  dCl_del/1 -> Add1/1
  dCl_der/1 -> Add1/2
  Add1/1 -> Gain1/1
  Add2/1 -> Gain2/1
  dCn_del/1 -> Add2/1
  dCn_der/1 -> Add2/2
  dCn_drl/1 -> Add3/1
  dCn_drr/1 -> Add3/2
  dCL_dAoA/1 -> Mux/1  "dCL_dAoA"
  dCm_dAoA/1 -> Mux/2  "dCm_dAoA"
  Gain/1 -> Mux/3  "dCm_de"
  Clb0/1 -> Mux/4  "Clb0"
  Gain1/1 -> Mux/5  "dCl_da"
  Cnb0/1 -> Mux/6  "Cnb0"
  Gain2/1 -> Mux/7  "dCn_da"
  Add3/1 -> Mux/8  "dCn_dr"
  Mux/1 -> coeff_deriv/1
  Add4/1 -> CL/1
  CLb/1 -> Add4/4
  CLel/1 -> Add4/2
  CL0/1 -> Add4/1
  CLer/1 -> Add4/3
  Selector5/1 -> Prelookup6/1  "delta_b"
  Prelookup6/1 -> CLb/2
  Prelookup5/1 -> dCn_drr/2
  Prelookup4/1 -> dCn_drl/2
  Prelookup3/1 -> dCn_der/2, dCl_der/2, CLer/2, dCm_der/2
  Prelookup2/1 -> dCl_del/2, dCn_del/2, CLel/2, dCm_del/2
  Abs1/1 -> Saturation3/1
  Selector1/1 -> Sign1/1, Abs1/1
  Sign1/1 -> Product1/1
  Saturation3/1 -> Product1/2
  Product1/1 -> Prelookup2/1  "delta_el"
  Sign/1 -> Product/1
  Saturation2/1 -> Product/2
  Abs/1 -> Saturation2/1
  Selector2/1 -> Sign/1, Abs/1
  Product/1 -> Prelookup3/1  "delta_er"
  Saturation1/1 -> Prelookup4/1  "delta_rl"
  Saturation/1 -> Prelookup5/1  "delta_rr"

== system simulator/Guidance System/Aero Coefficients ==
  AoA : Inport
  M : Inport  Port=2
  delta_b : Inport  Port=3
  Add : Sum
  Add1 : Sum
  AoA Table : PreLookup  BreakpointsData=simdb.aero.AoA_table  OutputSelection=Index and fraction as bus  BeginIndexSearchUsingPreviousIndexResult=on  ExtrapMethod=Linear  RemoveProtectionInput=on
  CD0 : Interpolation_n-D  Table=simdb.aero.CD0  RequireIndexFractionAsBus=on  RemoveProtectionIndex=on  InternalRulePriority=Speed
      settings: InputPortMap=u0,u1
  CDb : Interpolation_n-D  NumberOfTableDimensions=3  Table=simdb.aero.CDb  RequireIndexFractionAsBus=on  RemoveProtectionIndex=on  InternalRulePriority=Speed
      settings: InputPortMap=u0,u1,u2
  CL0 : Interpolation_n-D  Table=simdb.aero.CL0  RequireIndexFractionAsBus=on  RemoveProtectionIndex=on  InternalRulePriority=Speed
      settings: InputPortMap=u0,u1
  CLb : Interpolation_n-D  NumberOfTableDimensions=3  Table=simdb.aero.CLb  RequireIndexFractionAsBus=on  RemoveProtectionIndex=on  InternalRulePriority=Speed
      settings: InputPortMap=u0,u1,u2
  M Table : PreLookup  BreakpointsData=simdb.aero.M_table  OutputSelection=Index and fraction as bus  BeginIndexSearchUsingPreviousIndexResult=on  ExtrapMethod=Linear  RemoveProtectionInput=on
  Mux : Mux
  Radians to Degrees : simulink_extras/Transformations/Radians to Degrees
  dCD_dAoA : Interpolation_n-D  Table=simdb.aero.dCD_dAoA  RequireIndexFractionAsBus=on  RemoveProtectionIndex=on  InternalRulePriority=Speed
      settings: InputPortMap=u0,u1
  dCL_dAoA : Interpolation_n-D  Table=simdb.aero.dCL_dAoA  RequireIndexFractionAsBus=on  RemoveProtectionIndex=on  InternalRulePriority=Speed
      settings: InputPortMap=u0,u1
  delta_b Table : PreLookup  BreakpointsData=simdb.aero.delta_b_table  OutputSelection=Index and fraction as bus  BeginIndexSearchUsingPreviousIndexResult=on  ExtrapMethod=Linear  RemoveProtectionInput=on
  coeffs : Outport
  wires:
  Add/1 -> Mux/1  "CD"
  Add1/1 -> Mux/2  "CL"
  AoA/1 -> Radians to Degrees/1
  Radians to Degrees/1 -> AoA Table/1
  M/1 -> M Table/1
  delta_b/1 -> delta_b Table/1
  AoA Table/1 -> dCL_dAoA/1, dCD_dAoA/1, CLb/1, CDb/1, CL0/1, CD0/1
  delta_b Table/1 -> CDb/2, CLb/2
  M Table/1 -> CD0/2, dCL_dAoA/2, dCD_dAoA/2, CLb/3, CDb/3, CL0/2
  CD0/1 -> Add/1
  CDb/1 -> Add/2
  CL0/1 -> Add1/1
  CLb/1 -> Add1/2
  dCD_dAoA/1 -> Mux/3  "dCD_dAoA"
  dCL_dAoA/1 -> Mux/4  "dCL_dAoA"
  Mux/1 -> coeffs/1

== system simulator/Guidance System/Bank Angle Limiter ==
  u : Inport
  Abs : Abs  SaturateOnIntegerOverflow=off
  Product1 : Product
  Saturation : Saturate  UpperLimit=deg2rad(165)  LowerLimit=deg2rad(2)
  Sign : Signum
  u_lim : Outport
  wires:
  Abs/1 -> Saturation/1
  Saturation/1 -> Product1/2
  Sign/1 -> Product1/1
  u/1 -> Sign/1, Abs/1
  Product1/1 -> u_lim/1

== system simulator/Guidance System/Density Derivative ==
  rho : Inport
  R : Inport  Port=2
  Delay One Step : Delay  DelayLength=1
  Delay One Step1 : Delay  DelayLength=1
  Product : Product  Inputs=*/
  Sum : Sum  Inputs=|+-
  Sum1 : Sum  Inputs=|+-
  drho_dR : Outport
  wires:
  rho/1 -> Sum/1
  Sum/1 -> Product/1, Delay One Step/1
  Delay One Step1/1 -> Sum1/2
  Delay One Step/1 -> Sum/2
  Sum1/1 -> Product/2, Delay One Step1/1
  R/1 -> Sum1/1
  Product/1 -> drho_dR/1

== system simulator/Guidance System/Reference Trajectory ==
  t : Inport
  M : Inport  Port=2
  Ref Angle of Attack : MATLAB Function  TreatAsAtomicUnit=on
  Ref Bank Angle : Lookup_n-D  NumberOfTableDimensions=1  BreakpointsForDimension1=gui.t_gui  BreakpointsForDimension2=[1:3]  Table=gui.u_gui(1,:)  RemoveProtectionInput=on  InternalRulePriority=Speed  RndMeth=Simplest
  Ref Trajectory : Subsystem
  Ref body flap deflection : Lookup_n-D  NumberOfTableDimensions=1  BreakpointsForDimension1=gui.t_gui  BreakpointsForDimension2=[1:3]  Table=gui.u_gui(2,:)  RemoveProtectionInput=on  InternalRulePriority=Speed  RndMeth=Simplest
  y_ref : Outport
  bank_ang_ref : Outport  Port=2
  delta_b_ref : Outport  Port=3
  AoA_ref : Outport  Port=4
  wires:
  Ref body flap deflection/1 -> delta_b_ref/1
  t/1 -> Ref Trajectory/1(t), Ref body flap deflection/1, Ref Bank Angle/1
  Ref Angle of Attack/1(AoA) -> AoA_ref/1
  Ref Bank Angle/1 -> bank_ang_ref/1
  M/1 -> Ref Angle of Attack/1(M)
  Ref Trajectory/1(y_ref) -> y_ref/1

== system simulator/Guidance System/Subsystem ==
  delta_cmd : Inport
  u_ref : Inport  Port=2
  AoA_ref : Inport  Port=3
  Add : Sum
  Add1 : Sum
  Saturation : Saturate  UpperLimit=deg2rad(42.5)  LowerLimit=deg2rad(0)
  Saturation1 : Saturate  UpperLimit=deg2rad(170)  LowerLimit=-deg2rad(170)
  Selector : Selector  InputPortWidth=2  IndexOptions=Index vector (dialog)  Indices=2  OutputSizes=1
  Selector1 : Selector  InputPortWidth=2  IndexOptions=Index vector (dialog)  Indices=1  OutputSizes=1
  bank_ang_cmd : Outport
  AoA_cmd : Outport  Port=2
  wires:
  Add/1 -> Saturation1/1
  Selector/1 -> Add/2
  u_ref/1 -> Add/1
  delta_cmd/1 -> Selector/1, Selector1/1
  Selector1/1 -> Add1/1
  AoA_ref/1 -> Add1/2
  Add1/1 -> Saturation/1
  Saturation/1 -> AoA_cmd/1
  Saturation1/1 -> bank_ang_cmd/1

== system simulator/Navigation System/Extended Kalman Filter ==
  x_prev : Inport
  P_prev : Inport  Port=2
  z_meas : Inport  Port=3
  dt : Inport  Port=4
  Add : Sum
  Covariance Matrix Estimation : Subsystem
  Covariance Matrix Update : Subsystem
  Kalman Gain : Subsystem
  Matrix Multiply : Product  Multiplication=Matrix(*)
  Rate Transition : RateTransition  InitialCondition=simdb.nav.x0  OutPortSampleTime=simdb.nav.tsamp
  Rate Transition1 : RateTransition  InitialCondition=simdb.nav.P0  OutPortSampleTime=simdb.nav.tsamp
  Subtract : Sum  Inputs=+-
  estimation function : MATLAB Function  TreatAsAtomicUnit=on  mask{mu=simdb.env.mu, K=simdb.nav.dq_K}
      mask prompts: mu "Gravitational parameter [m^3/s^2]:"; K "dq integration gain:"
  estimation matrix : MATLAB Function  TreatAsAtomicUnit=on  mask{mu=simdb.env.mu}
      mask prompts: mu "Gravitational parameter [m^2/s^2]:"
  observation function : MATLAB Function  TreatAsAtomicUnit=on  mask{Ma=simdb.nav.Ma, Mo=simdb.nav.Mo}
      mask prompts: Ma "Acc Misalignment Matrix:"; Mo "Gyr Misalignment Matrix:"
  observation matrix : MATLAB Function  TreatAsAtomicUnit=on  mask{Ma=simdb.nav.Ma, Mo=simdb.nav.Mo}
      mask prompts: Ma "Acc Misalignment Matrix:"; Mo "Gyr Misalignment Matrix:"
  x_new : Outport
  P_new : Outport  Port=2
  wires:
  dt/1 -> observation function/2(dt), observation matrix/2(dt), estimation function/2(dt)
  x_prev/1 -> estimation matrix/1(x), estimation function/1(x)
  observation function/1(z) -> Subtract/2  "z_est"
  estimation function/1(x_est) -> Add/1, observation matrix/1(x), observation function/1(x)  "x_est"
  observation matrix/1(H) -> Covariance Matrix Update/2(H), Kalman Gain/1(H)
  Kalman Gain/1(K) -> Matrix Multiply/1, Covariance Matrix Update/1(K)
  z_meas/1 -> Subtract/1
  Subtract/1 -> Matrix Multiply/2
  Matrix Multiply/1 -> Add/2
  P_prev/1 -> Covariance Matrix Estimation/2(P_prev)
  Covariance Matrix Estimation/1(P_est) -> Covariance Matrix Update/3(P_est), Kalman Gain/2(P_est)
  Covariance Matrix Update/1(P_new) -> Rate Transition1/1
  Add/1 -> Rate Transition/1
  estimation matrix/1(F) -> Covariance Matrix Estimation/1(F)
  Rate Transition/1 -> x_new/1
  Rate Transition1/1 -> P_new/1

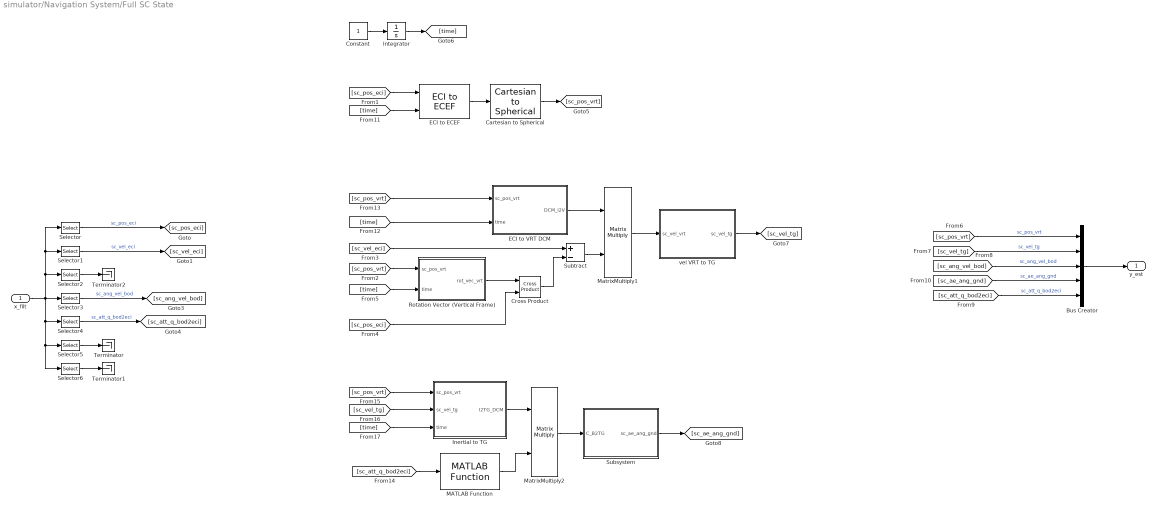
== system simulator/Navigation System/Full SC State ==
  x_filt : Inport
  Bus Creator : BusCreator  Inputs=5
  Cartesian to Spherical : sim_lib/Cartesian to Spherical  SystemSampleTime=-1  VariantActivationTime=update diagram  Latency=0  AutoFrameSizeCalculation=off
  Constant : Constant
  Cross Product : matrix_library/Cross Product
  ECI to ECEF : sim_lib/ECI to ECEF  omega_cb=0
  ECI to VRT DCM : Subsystem
  Inertial to TG : Subsystem
  Integrator : Integrator
  MATLAB Function : sim_lib/MATLAB Function  SystemSampleTime=-1  VariantActivationTime=update diagram  Latency=0  AutoFrameSizeCalculation=off
      settings: LibrarySourceBlock=|
      | simulink/User-Defined
      | Functions/MATLAB Function
  MatrixMultiply1 : Product  Multiplication=Matrix(*)
  MatrixMultiply2 : Product  Multiplication=Matrix(*)
  Rotation Vector (Vertical Frame) : Subsystem
  Selector : Selector  InputPortWidth=22  IndexOptions=Index vector (dialog)  Indices=[1 2 3]  OutputSizes=1
  Selector1 : Selector  InputPortWidth=22  IndexOptions=Index vector (dialog)  Indices=[4 5 6]  OutputSizes=1
  Selector2 : Selector  InputPortWidth=22  IndexOptions=Index vector (dialog)  Indices=[7 8 9]  OutputSizes=1
  Selector3 : Selector  InputPortWidth=22  IndexOptions=Index vector (dialog)  Indices=[10 11 12]  OutputSizes=1
  Selector4 : Selector  InputPortWidth=22  IndexOptions=Index vector (dialog)  Indices=[13 14 15 16]  OutputSizes=1
  Selector5 : Selector  InputPortWidth=22  IndexOptions=Index vector (dialog)  Indices=[17 18 19]  OutputSizes=1
  Selector6 : Selector  InputPortWidth=22  IndexOptions=Index vector (dialog)  Indices=[20 21 22]  OutputSizes=1
  Subsystem : Subsystem
  Subtract : Sum  Inputs=+-
  Terminator : Terminator
  Terminator1 : Terminator
  Terminator2 : Terminator
  vel VRT to TG : Subsystem
  y_est : Outport
  wires:
  x_filt/1 -> Selector2/1, Selector1/1, Selector/1, Selector6/1, Selector5/1, Selector4/1, Selector3/1
  Selector1/1 -> [sc_vel_eci]  "sc_vel_eci"
  Selector3/1 -> [sc_ang_vel_bod]  "sc_ang_vel_bod"
  Selector4/1 -> [sc_att_q_bod2eci]  "sc_att_q_bod2eci"
  Selector5/1 -> Terminator/1
  Selector6/1 -> Terminator1/1
  Bus Creator/1 -> y_est/1
  Selector/1 -> [sc_pos_eci]  "sc_pos_eci"
  [sc_pos_vrt] -> Bus Creator/1  "sc_pos_vrt"
  [sc_vel_tg] -> Bus Creator/2  "sc_vel_tg"
  [sc_ang_vel_bod] -> Bus Creator/3  "sc_ang_vel_bod"
  [sc_att_q_bod2eci] -> Bus Creator/5  "sc_att_q_bod2eci"
  [sc_ae_ang_gnd] -> Bus Creator/4  "sc_ae_ang_gnd"
  ECI to ECEF/1 -> Cartesian to Spherical/1
  [sc_pos_eci] -> ECI to ECEF/1
  Cartesian to Spherical/1 -> [sc_pos_vrt]
  Constant/1 -> Integrator/1
  Integrator/1 -> [time]
  [time] -> Rotation Vector (Vertical Frame)/2(time)
  [time] -> ECI to ECEF/2
  [sc_pos_vrt] -> Rotation Vector (Vertical Frame)/1(sc_pos_vrt)
  Rotation Vector (Vertical Frame)/1(rot_vec_vrt) -> Cross Product/1
  [sc_pos_eci] -> Cross Product/2
  [sc_vel_eci] -> Subtract/1
  Cross Product/1 -> Subtract/2
  Subtract/1 -> MatrixMultiply1/2
  ECI to VRT DCM/1(DCM_I2V) -> MatrixMultiply1/1
  [time] -> ECI to VRT DCM/2(time)
  [sc_pos_vrt] -> ECI to VRT DCM/1(sc_pos_vrt)
  MatrixMultiply1/1 -> vel VRT to TG/1(sc_vel_vrt)
  vel VRT to TG/1(sc_vel_tg) -> [sc_vel_tg]
  [sc_att_q_bod2eci] -> MATLAB Function/1
  [sc_pos_vrt] -> Inertial to TG/1(sc_pos_vrt)
  [sc_vel_tg] -> Inertial to TG/2(sc_vel_tg)
  [time] -> Inertial to TG/3(time)
  Inertial to TG/1(I2TG_DCM) -> MatrixMultiply2/1
  MATLAB Function/1 -> MatrixMultiply2/2
  MatrixMultiply2/1 -> Subsystem/1(C_B2TG)
  Subsystem/1(sc_ae_ang_gnd) -> [sc_ae_ang_gnd]
  Selector2/1 -> Terminator2/1
